simulink model "Bode_plots_time_delay"  (R2020a)
settings: Solver=VariableStepAuto  StartTime=0.0  StopTime=step_time  RelTol=1e-10
values from neighbouring files (symbols this model uses):
  K = K_vec(i)    [Bode_plots_time_delay.m]    (also in Time_delay_system.m = 3; Time_delay_system_2.m = 3)
  Kc = Kc_vec(i)    [Bode_plots_time_delay.m]
  tau = 300    [Bode_plots_time_delay.m]
settings Model: Creator=sangmin  LastModifiedBy=sangmin
settings DataIOCC: ReturnWorkspaceOutputs=off

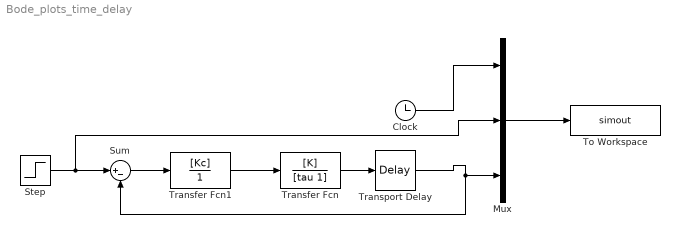
== system Bode_plots_time_delay ==
  Clock : Clock
  Mux : Mux  Inputs=3
  Step : Step  Time=1800  Before=2  After=3  SampleTime=0
  Sum : Sum  Inputs=|+-
  To Workspace : ToWorkspace  VariableName=simout  SampleTime=-1
  Transfer Fcn : TransferFcn  Numerator=[K]  Denominator=[tau 1]
  Transfer Fcn1 : TransferFcn  Numerator=[Kc]  Denominator=[1]
  Transport Delay : TransportDelay  DelayTime=120
  wires:
  Transport Delay/1 -> Mux/3, Sum/2
  Transfer Fcn/1 -> Transport Delay/1
  Transfer Fcn1/1 -> Transfer Fcn/1
  Sum/1 -> Transfer Fcn1/1
  Step/1 -> Mux/2, Sum/1
  Clock/1 -> Mux/1
  Mux/1 -> To Workspace/1
